simulink model "emit"  (R2019b)
settings: Solver=VariableStepAuto  StartTime=0.0  StopTime=10.0  RelTol=1e-3
InitFcn:
  | Samplesperframe=512;
  | Sampling_time=1/20e6;
  | RFactor=0.25;
  | Upsmp=8;
  | M=16;
  | 
  | global k;
  | k=4;
  | global q;
  | q=1;
  | global minq;
  | minq = min(q,10);%延时项最大为10
  | 
  | global a;
  | global even;
  | even = 0; %1或0
  | global d;
  | if even == 1 %包含奇偶次项
  | a=eye((k*(minq+1)),1);
  | d=1;
  | else if even == 0 %只包含奇次项
  | a=eye(fix((k+1)/2)*(minq+1),1);
  | d=2;
  | end
  | end
libraries: commfilt2 x1, commrandsrc3 x1, commdigbbndam3 x1
settings Model: Creator=noether  LastModifiedBy=苗一依

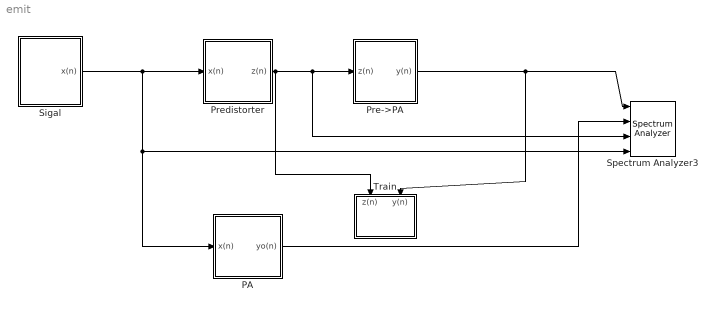
== system emit ==
  PA : Subsystem
  Pre->PA : Subsystem
  Predistorter : Subsystem
  Sigal : Subsystem
  Spectrum Analyzer3 : SpectrumAnalyzer  NumInputPorts=4
  Train : Subsystem
  wires:
  PA/1(yo(n)) -> Spectrum Analyzer3/2
  Sigal/1(x(n)) -> PA/1(x(n)), Spectrum Analyzer3/4, Predistorter/1(x(n))
  Predistorter/1(z(n)) -> Train/1(z(n)), Spectrum Analyzer3/3, Pre->PA/1(z(n))
  Pre->PA/1(y(n)) -> Train/2(y(n)), Spectrum Analyzer3/1

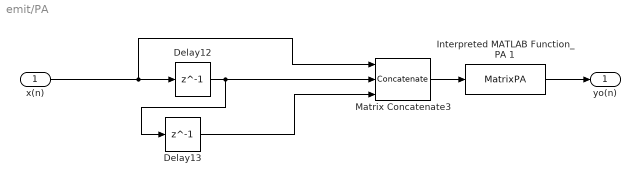
== system emit/PA ==
  x(n) : Inport
  Delay12 : Delay  DelayLength=1  InputProcessing=Columns as channels (frame based)
  Delay13 : Delay  DelayLength=1  InputProcessing=Columns as channels (frame based)
  Interpreted MATLAB Function_PA 1 : MATLABFcn  MATLABFcn=MatrixPA
  Matrix Concatenate3 : Concatenate  NumInputs=3  Mode=Multidimensional array  ConcatenateDimension=2
  yo(n) : Outport
  wires:
  x(n)/1 -> Matrix Concatenate3/1, Delay12/1
  Delay13/1 -> Matrix Concatenate3/3
  Matrix Concatenate3/1 -> Interpreted MATLAB Function_PA 1/1
  Delay12/1 -> Delay13/1, Matrix Concatenate3/2
  Interpreted MATLAB Function_PA 1/1 -> yo(n)/1

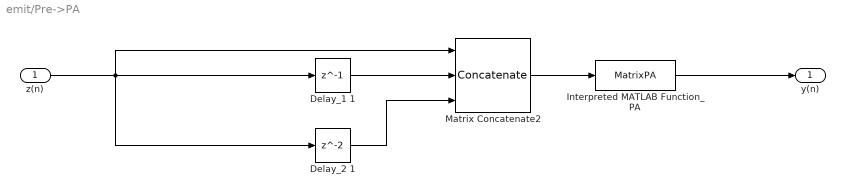
== system emit/Pre->PA ==
  z(n) : Inport
  Delay_1 1 : Delay  DelayLength=1  InputProcessing=Columns as channels (frame based)
  Delay_2 1 : Delay  InputProcessing=Columns as channels (frame based)
  "Interpreted MATLAB Function_PA " : MATLABFcn  MATLABFcn=MatrixPA
  Matrix Concatenate2 : Concatenate  NumInputs=3  Mode=Multidimensional array  ConcatenateDimension=2
  y(n) : Outport
  wires:
  Matrix Concatenate2/1 -> "Interpreted MATLAB Function_PA "/1
  Delay_1 1/1 -> Matrix Concatenate2/2
  Delay_2 1/1 -> Matrix Concatenate2/3
  z(n)/1 -> Matrix Concatenate2/1, Delay_2 1/1, Delay_1 1/1
  "Interpreted MATLAB Function_PA "/1 -> y(n)/1

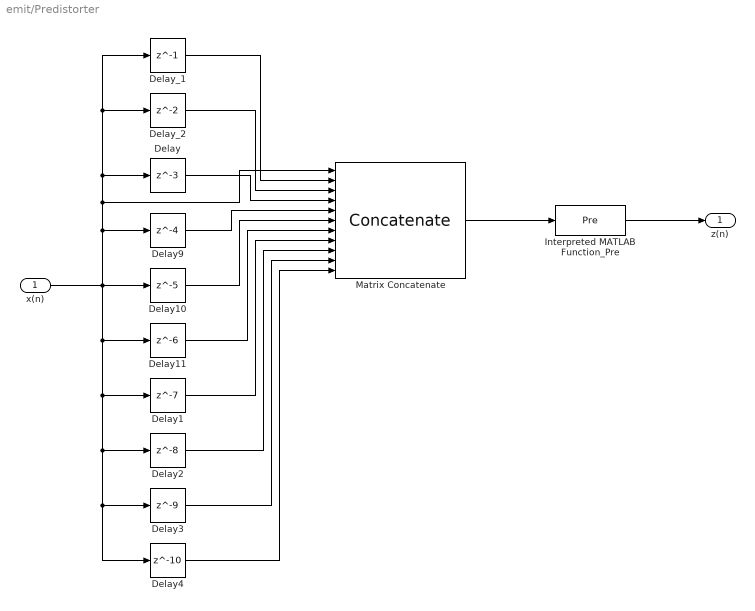
== system emit/Predistorter ==
  x(n) : Inport
  Delay : Delay  DelayLength=3  InputProcessing=Columns as channels (frame based)
  Delay1 : Delay  DelayLength=7  InputProcessing=Columns as channels (frame based)
  Delay10 : Delay  DelayLength=5  InputProcessing=Columns as channels (frame based)
  Delay11 : Delay  DelayLength=6  InputProcessing=Columns as channels (frame based)
  Delay2 : Delay  DelayLength=8  InputProcessing=Columns as channels (frame based)
  Delay3 : Delay  DelayLength=9  InputProcessing=Columns as channels (frame based)
  Delay4 : Delay  DelayLength=10  InputProcessing=Columns as channels (frame based)
  Delay9 : Delay  DelayLength=4  InputProcessing=Columns as channels (frame based)
  "Delay_1 " : Delay  DelayLength=1  InputProcessing=Columns as channels (frame based)
  "Delay_2 " : Delay  InputProcessing=Columns as channels (frame based)
  Interpreted MATLAB Function_Pre : MATLABFcn  MATLABFcn=Pre
  Matrix Concatenate : Concatenate  NumInputs=11  Mode=Multidimensional array  ConcatenateDimension=2
  z(n) : Outport
  wires:
  x(n)/1 -> Delay4/1, Delay3/1, Delay2/1, Delay1/1, Delay11/1, "Delay_1 "/1, "Delay_2 "/1, Delay/1, Matrix Concatenate/1, Delay9/1, Delay10/1
  Matrix Concatenate/1 -> Interpreted MATLAB Function_Pre/1
  "Delay_2 "/1 -> Matrix Concatenate/3
  Delay/1 -> Matrix Concatenate/4
  Delay10/1 -> Matrix Concatenate/6
  "Delay_1 "/1 -> Matrix Concatenate/2
  Delay9/1 -> Matrix Concatenate/5
  Delay11/1 -> Matrix Concatenate/7
  Interpreted MATLAB Function_Pre/1 -> z(n)/1
  Delay1/1 -> Matrix Concatenate/8
  Delay2/1 -> Matrix Concatenate/9
  Delay3/1 -> Matrix Concatenate/10
  Delay4/1 -> Matrix Concatenate/11

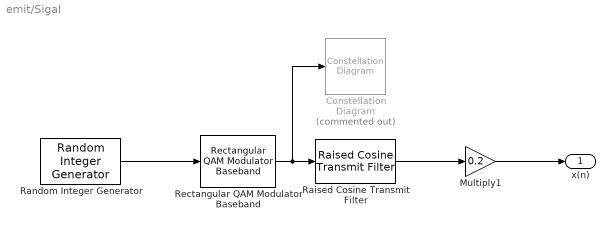
== system emit/Sigal ==
  Constellation Diagram : ConstellationDiagram  Commented=on
  Multiply1 : Gain  Gain=0.2
  Raised Cosine Transmit Filter : commfilt2/Raised Cosine Transmit Filter  filtType=Square root  R=RFactor  filtSpan=50  N=8  filterGain=1  InputProcessing=Columns as channels (frame based)  RateOptions=Enforce single-rate processing  framing=Mute  checkCoeff=off  variableName=rcTxFilt  checkGain=Normalized  sampMode=Mute  saveAsFlag=0  currentFiltSpan=50  D=(50)/2  launchFVT=on  roundingMode=Floor  overflowMode=off  coeffDataTypeStr=Inherit: Same word length as input  coeffMin=[]  coeffMax=[]  coeffLastDataTypeStr=Inherit: Same word length as input  outputDataTypeStr=Inherit: Same as accumulator  outputMin=[]  outputMax=[]  outputLastDataTypeStr=Inherit: Same as accumulator
      settings: SourceProductName=Communications Toolbox
  Random Integer Generator : commrandsrc3/Random Integer Generator  SetSize=M  SeedSource=Parameter  Seed=10  SampleTime=Sampling_time  SamplesPerFrame=Samplesperframe  OutputDataType=double  SimulateUsing=Interpreted execution
      settings: SourceProductName=Communications Toolbox
  Rectangular QAM Modulator Baseband : commdigbbndam3/Rectangular QAM Modulator Baseband  M=M  InType=Integer  Enc=Gray  Mapping=[0:15]  PowType=Min. distance between symbols  MinDist=2  AvgPow=1  PeakPow=1  Ph=0  outDtype=double  outWordLen=16  outUDDataType=sfix(16)  outFracLenMode=Best precision  outFracLen=15  outDataTypeStr=double  outLastDataTypeStr=double
      settings: SourceProductName=Communications Toolbox
  x(n) : Outport
  wires:
  Raised Cosine Transmit Filter/1 -> Multiply1/1
  Random Integer Generator/1 -> Rectangular QAM Modulator Baseband/1
  Rectangular QAM Modulator Baseband/1 -> Constellation Diagram/1, Raised Cosine Transmit Filter/1
  Multiply1/1 -> x(n)/1

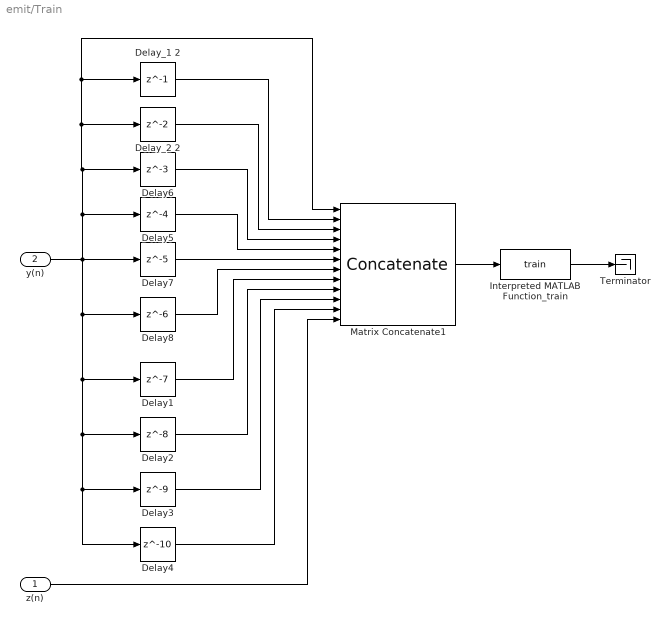
== system emit/Train ==
  z(n) : Inport
  y(n) : Inport  Port=2
  Delay1 : Delay  DelayLength=7  InputProcessing=Columns as channels (frame based)
  Delay2 : Delay  DelayLength=8  InputProcessing=Columns as channels (frame based)
  Delay3 : Delay  DelayLength=9  InputProcessing=Columns as channels (frame based)
  Delay4 : Delay  DelayLength=10  InputProcessing=Columns as channels (frame based)
  Delay5 : Delay  DelayLength=4  InputProcessing=Columns as channels (frame based)
  Delay6 : Delay  DelayLength=3  InputProcessing=Columns as channels (frame based)
  Delay7 : Delay  DelayLength=5  InputProcessing=Columns as channels (frame based)
  Delay8 : Delay  DelayLength=6  InputProcessing=Columns as channels (frame based)
  Delay_1 2 : Delay  DelayLength=1  InputProcessing=Columns as channels (frame based)
  Delay_2 2 : Delay  InputProcessing=Columns as channels (frame based)
  Interpreted MATLAB Function_train : MATLABFcn  MATLABFcn=train
  Matrix Concatenate1 : Concatenate  NumInputs=12  Mode=Multidimensional array  ConcatenateDimension=2
  Terminator : Terminator
  wires:
  Delay5/1 -> Matrix Concatenate1/5
  Interpreted MATLAB Function_train/1 -> Terminator/1
  Delay8/1 -> Matrix Concatenate1/7
  Delay7/1 -> Matrix Concatenate1/6
  Delay6/1 -> Matrix Concatenate1/4
  Delay_1 2/1 -> Matrix Concatenate1/2
  Delay_2 2/1 -> Matrix Concatenate1/3
  Matrix Concatenate1/1 -> Interpreted MATLAB Function_train/1
  y(n)/1 -> Delay8/1, Delay1/1, Delay2/1, Delay3/1, Delay4/1, Matrix Concatenate1/1, Delay_1 2/1, Delay_2 2/1, Delay6/1, Delay5/1, Delay7/1
  Delay1/1 -> Matrix Concatenate1/8
  Delay2/1 -> Matrix Concatenate1/9
  Delay3/1 -> Matrix Concatenate1/10
  Delay4/1 -> Matrix Concatenate1/11
  z(n)/1 -> Matrix Concatenate1/12
